simulink model "student_model_ref"  (Simulink 7.5)
settings: Solver=ode45  StartTime=0.0  StopTime=t_sim  RelTol=1e-3
values from neighbouring files (symbols this model uses):
  A = [0 1; -wn_model^2 -2*zeta_model*wn_model]    [student_lab4_model_ref.m]
  Ap = [0 1; -wn^2 -2*zeta*wn]    [student_lab4_model_ref.m]
  B = [0; 1]    [student_lab4_model_ref.m]
  Bp = [0; 1]    [student_lab4_model_ref.m]
  C = eye(2)    [student_lab4_model_ref.m]
  Cp = eye(2)    [student_lab4_model_ref.m]
  D = [0;0]    [student_lab4_model_ref.m]
  Dp = [0;0]    [student_lab4_model_ref.m]
  step1 = v_step    (= 0.243)    [student_lab4_model_ref.m]
  step2 = -v_step    (= -0.243)    [student_lab4_model_ref.m]
  t_off = 5    [student_lab4_model_ref.m]
  t_on = 1    [student_lab4_model_ref.m]
undefined symbols (not defined in the file or in its folder): student_model_ref_controller
settings Model: Creator=Kelvin  LastModifiedBy=Kelvin

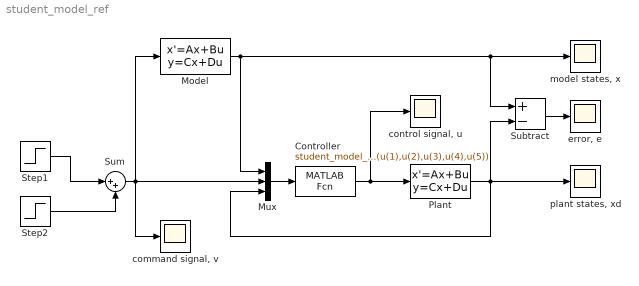
== system student_model_ref ==
  Controller : MATLABFcn  MATLABFcn=student_model_ref_controller(u(1),u(2),u(3),u(4),u(5))
  Model : StateSpace  A=A  B=B  C=C  D=D
  Mux : Mux  Inputs=3
  Plant : StateSpace  A=Ap  B=Bp  C=Cp  D=Dp
  Step1 : Step  Time=t_on  After=step1  SampleTime=0  ZeroCross=off
  Step2 : Step  Time=t_off  After=step2  SampleTime=0  ZeroCross=off
  Subtract : Sum  Inputs=+-  OutDataType=fixdt(1, 16)  OutScaling=2^-10
  Sum : Sum  Inputs=|++  OutDataType=fixdt(1, 16)  OutScaling=2^0
  "command signal, v" : Scope
      settings: SaveName=ScopeData4
  "control signal, u" : Scope
      settings: TimeRange=10  YMin=0  YMax=0.35  SaveName=ScopeData3
  "error, e" : Scope
      settings: SaveName=ScopeData2
  "model states, x" : Scope
      settings: TimeRange=10  YMin=0  YMax=0.02
  "plant states, xd" : Scope
      settings: TimeRange=10  YMin=-0.005  YMax=0.02
  wires:
  Sum/1 -> Model/1, Mux/2, "command signal, v"/1
  Mux/1 -> Controller/1
  Controller/1 -> "control signal, u"/1, Plant/1
  Plant/1 -> Mux/3, "plant states, xd"/1, Subtract/2
  Model/1 -> Mux/1, Subtract/1, "model states, x"/1
  Subtract/1 -> "error, e"/1
  Step1/1 -> Sum/1
  Step2/1 -> Sum/2
